simulink model "Clarke_Concordia"  (R2018b)
settings: Solver=VariableStepAuto  StartTime=0.0  StopTime=10.0  MaxStep=1/(fn*100)  MinStep=1/(fn*1000)  RelTol=1e-3
values from neighbouring files (symbols this model uses):
  A = sqrt(2/3)*[1 -0.5 -0.5; 0 sqrt(3)/2 -sqrt(3)/2; sqrt(0.5) sqrt(0.5) sqrt(0.5)]    [Comm_Vect.m]    (also in clarke_conc.m)
  fn = 50    [Comm_Vect.m]    (also in clarke_conc.m)
  Vn = 220    [Comm_Vect.m]    (also in clarke_conc.m)
settings Model: Creator=cindyiskandar  LastModifiedBy=cindyiskandar

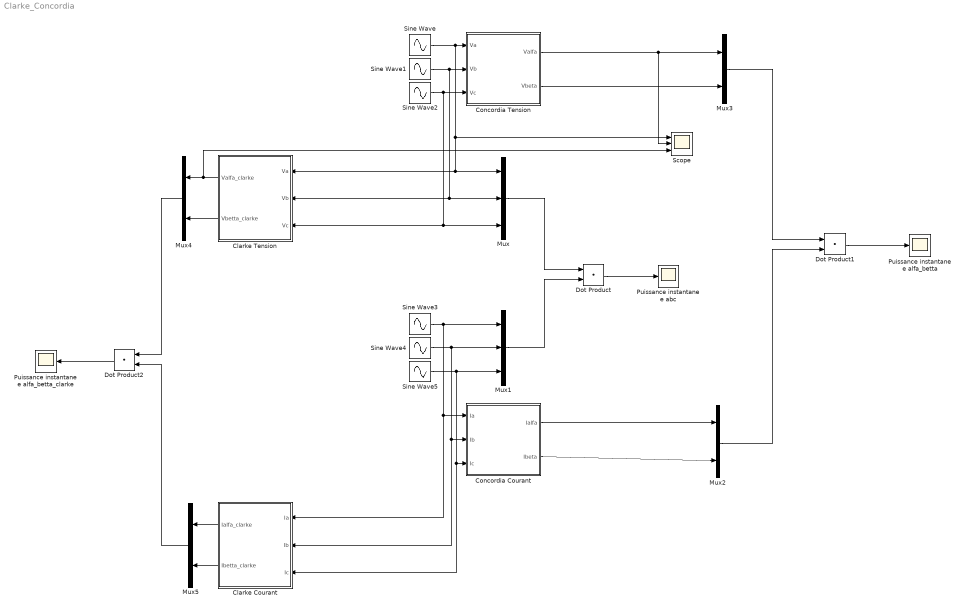
== system Clarke_Concordia ==
  Clarke Courant : Subsystem
  Clarke Tension : Subsystem
  Concordia Courant : Subsystem
  "Concordia Tension " : Subsystem
  Dot Product : DotProduct  InputSameDT=on  OutDataTypeStr=Inherit: Inherit via internal rule
  Dot Product1 : DotProduct  InputSameDT=on  OutDataTypeStr=Inherit: Inherit via internal rule
  Dot Product2 : DotProduct  InputSameDT=on  OutDataTypeStr=Inherit: Inherit via internal rule
  Mux : Mux  Inputs=3
  Mux1 : Mux  Inputs=3
  Mux{2..5} (4 alike) : Mux  Inputs=2
  Puissance instantanee alfa_betta : Scope
  Puissance instantanee alfa_betta_clarke : Scope
  Puissance instantanee abc : Scope
  Scope : Scope  NumInputPorts=3
  Sine Wave : Sin  Amplitude=Vn  Frequency=2*pi*fn  SampleTime=0
  Sine Wave1 : Sin  Amplitude=Vn  Frequency=2*pi*fn  Phase=2*pi/3  SampleTime=0
  Sine Wave2 : Sin  Amplitude=Vn  Frequency=2*pi*fn  Phase=4*pi/3  SampleTime=0
  Sine Wave3 : Sin  Amplitude=Vn  Frequency=2*pi*fn  SampleTime=0
  Sine Wave4 : Sin  Amplitude=Vn  Frequency=2*pi*fn  Phase=2*pi/3  SampleTime=0
  Sine Wave5 : Sin  Amplitude=Vn  Frequency=2*pi*fn  Phase=4*pi/3  SampleTime=0
  wires:
  Sine Wave/1 -> Mux/1, Clarke Tension/1(Va), Scope/1, "Concordia Tension "/1("Va ")
  Sine Wave1/1 -> Mux/2, Clarke Tension/2(Vb), "Concordia Tension "/2("Vb ")
  Sine Wave2/1 -> Mux/3, Clarke Tension/3(Vc), "Concordia Tension "/3(Vc)
  "Concordia Tension "/1(Valfa) -> Scope/2, Mux3/1
  "Concordia Tension "/2("Vbeta ") -> Mux3/2
  Mux/1 -> Dot Product/1
  Sine Wave3/1 -> Clarke Courant/1(Ia), Concordia Courant/1(Ia), Mux1/1
  Sine Wave4/1 -> Clarke Courant/2(Ib), Concordia Courant/2(Ib), Mux1/2
  Sine Wave5/1 -> Clarke Courant/3(Ic), Concordia Courant/3(Ic), Mux1/3
  Mux1/1 -> Dot Product/2
  Dot Product/1 -> Puissance instantanee abc/1
  Concordia Courant/1(Ialfa) -> Mux2/1
  Concordia Courant/2("Ibeta ") -> Mux2/2
  Dot Product1/1 -> Puissance instantanee alfa_betta/1
  Mux3/1 -> Dot Product1/1
  Mux2/1 -> Dot Product1/2
  Clarke Tension/2(Vbetta_clarke) -> Mux4/2
  Clarke Tension/1(Valfa_clarke) -> Scope/3, Mux4/1
  Clarke Courant/1(Ialfa_clarke) -> Mux5/1
  Clarke Courant/2(Ibetta_clarke) -> Mux5/2
  Dot Product2/1 -> Puissance instantanee alfa_betta_clarke/1
  Mux4/1 -> Dot Product2/1
  Mux5/1 -> Dot Product2/2

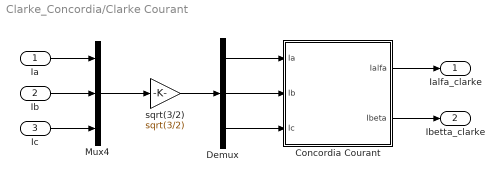
== system Clarke_Concordia/Clarke Courant ==
  Ia : Inport
  Ib : Inport  Port=2
  Ic : Inport  Port=3
  Concordia Courant : Subsystem
  Demux : Demux  Outputs=3
  Mux4 : Mux  Inputs=3
  sqrt(3/2) : Gain  Gain=sqrt(3/2)
  Ialfa_clarke : Outport
  Ibetta_clarke : Outport  Port=2
  wires:
  Ic/1 -> Mux4/3
  Demux/1 -> Concordia Courant/1(Ia)
  Ia/1 -> Mux4/1
  Concordia Courant/2("Ibeta ") -> Ibetta_clarke/1
  Demux/3 -> Concordia Courant/3(Ic)
  Demux/2 -> Concordia Courant/2(Ib)
  sqrt(3/2)/1 -> Demux/1
  Concordia Courant/1(Ialfa) -> Ialfa_clarke/1
  Mux4/1 -> sqrt(3/2)/1
  Ib/1 -> Mux4/2

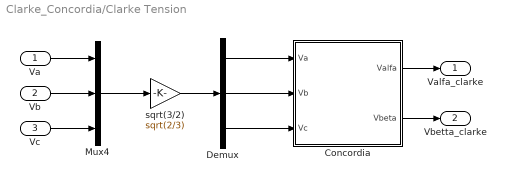
== system Clarke_Concordia/Clarke Tension ==
  Va : Inport
  Vb : Inport  Port=2
  Vc : Inport  Port=3
  "Concordia " : Subsystem
  Demux : Demux  Outputs=3
  Mux4 : Mux  Inputs=3
  sqrt(3/2) : Gain  Gain=sqrt(2/3)
  Valfa_clarke : Outport
  Vbetta_clarke : Outport  Port=2
  wires:
  Vc/1 -> Mux4/3
  Demux/1 -> "Concordia "/1("Va ")
  Va/1 -> Mux4/1
  "Concordia "/2("Vbeta ") -> Vbetta_clarke/1
  Demux/3 -> "Concordia "/3(Vc)
  Demux/2 -> "Concordia "/2("Vb ")
  sqrt(3/2)/1 -> Demux/1
  "Concordia "/1(Valfa) -> Valfa_clarke/1
  Mux4/1 -> sqrt(3/2)/1
  Vb/1 -> Mux4/2

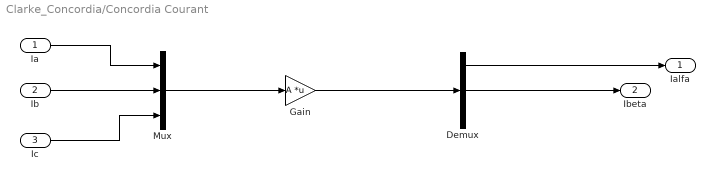
== system Clarke_Concordia/Concordia Courant ==
  Ia : Inport
  Ib : Inport  Port=2
  Ic : Inport  Port=3
  Demux : Demux  Outputs=3
  Gain : Gain  Gain=A  Multiplication=Matrix(K*u) (u vector)
  Mux : Mux  Inputs=3
  Ialfa : Outport
  "Ibeta " : Outport  Port=2
  wires:
  Demux/1 -> Ialfa/1
  Ia/1 -> Mux/1
  Mux/1 -> Gain/1
  Gain/1 -> Demux/1
  Ib/1 -> Mux/2
  Ic/1 -> Mux/3
  Demux/2 -> "Ibeta "/1

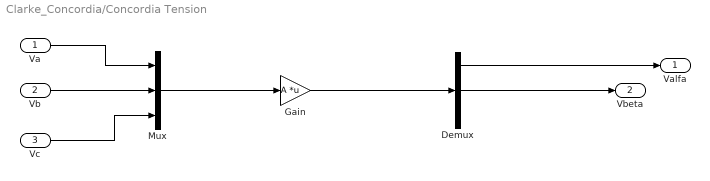
== system Clarke_Concordia/Concordia Tension  ==
  "Va " : Inport
  "Vb " : Inport  Port=2
  Vc : Inport  Port=3
  Demux : Demux  Outputs=3
  Gain : Gain  Gain=A  Multiplication=Matrix(K*u) (u vector)
  Mux : Mux  Inputs=3
  Valfa : Outport
  "Vbeta " : Outport  Port=2
  wires:
  Demux/1 -> Valfa/1
  "Va "/1 -> Mux/1
  Mux/1 -> Gain/1
  Gain/1 -> Demux/1
  "Vb "/1 -> Mux/2
  Vc/1 -> Mux/3
  Demux/2 -> "Vbeta "/1

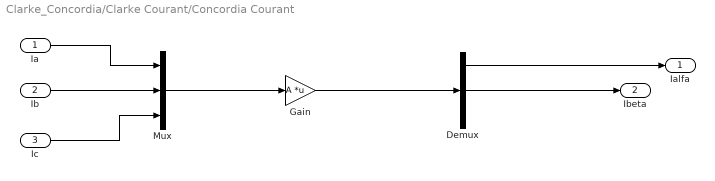
== system Clarke_Concordia/Clarke Courant/Concordia Courant ==
  Ia : Inport
  Ib : Inport  Port=2
  Ic : Inport  Port=3
  Demux : Demux  Outputs=3
  Gain : Gain  Gain=A  Multiplication=Matrix(K*u) (u vector)
  Mux : Mux  Inputs=3
  Ialfa : Outport
  "Ibeta " : Outport  Port=2
  wires:
  Demux/1 -> Ialfa/1
  Ia/1 -> Mux/1
  Mux/1 -> Gain/1
  Gain/1 -> Demux/1
  Ib/1 -> Mux/2
  Ic/1 -> Mux/3
  Demux/2 -> "Ibeta "/1

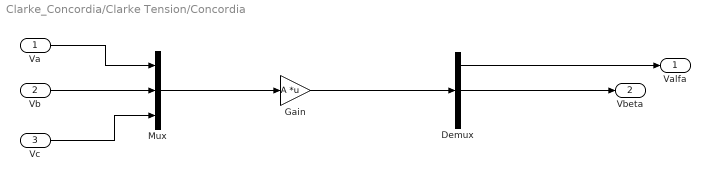
== system Clarke_Concordia/Clarke Tension/Concordia  ==
  "Va " : Inport
  "Vb " : Inport  Port=2
  Vc : Inport  Port=3
  Demux : Demux  Outputs=3
  Gain : Gain  Gain=A  Multiplication=Matrix(K*u) (u vector)
  Mux : Mux  Inputs=3
  Valfa : Outport
  "Vbeta " : Outport  Port=2
  wires:
  Demux/1 -> Valfa/1
  "Va "/1 -> Mux/1
  Mux/1 -> Gain/1
  Gain/1 -> Demux/1
  "Vb "/1 -> Mux/2
  Vc/1 -> Mux/3
  Demux/2 -> "Vbeta "/1
